simulink model "constant_volt"  (R2023b)
settings: Solver=VariableStepAuto  StartTime=0.0  StopTime=stepp.sim_time  RelTol=1e-3
values from neighbouring files (symbols this model uses):
  Bat =     [Samsung_30Q_18650_pack.mat]
undefined symbols (not defined in the file or in its folder): boost, ccm_m_op, ccm_reg_param, Ci, dcm_op, dcm_reg_param, Gp_ccm, Gp_dcm, Kr, m0_ccm, pv_data, pv_eq, Ramp, Ru, sim_op, stepp, Ti
libraries: spsSeriesRLCBranchLib x7, spsCurrentMeasurementLib x4, spsVoltageMeasurementLib x3, slpidlib x3, spsDiodeLib x1, spsControlledCurrentSourceLib x1, spsIdealSwitchLib x1, spsControlledVoltageSourceLib x1, simulink_extras x1, spsBistableLib x1, sps_lib x1
settings Model: Creator=teo  LastModifiedBy=teo
settings DataIOCC: ReturnWorkspaceOutputsName=CV_response

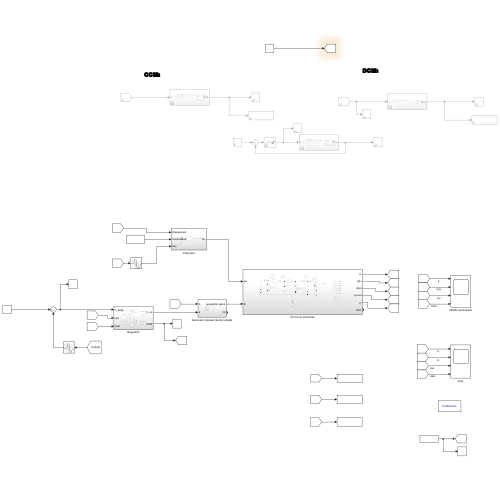
[thumbnail: Simulink's stored preview of the top-level diagram]
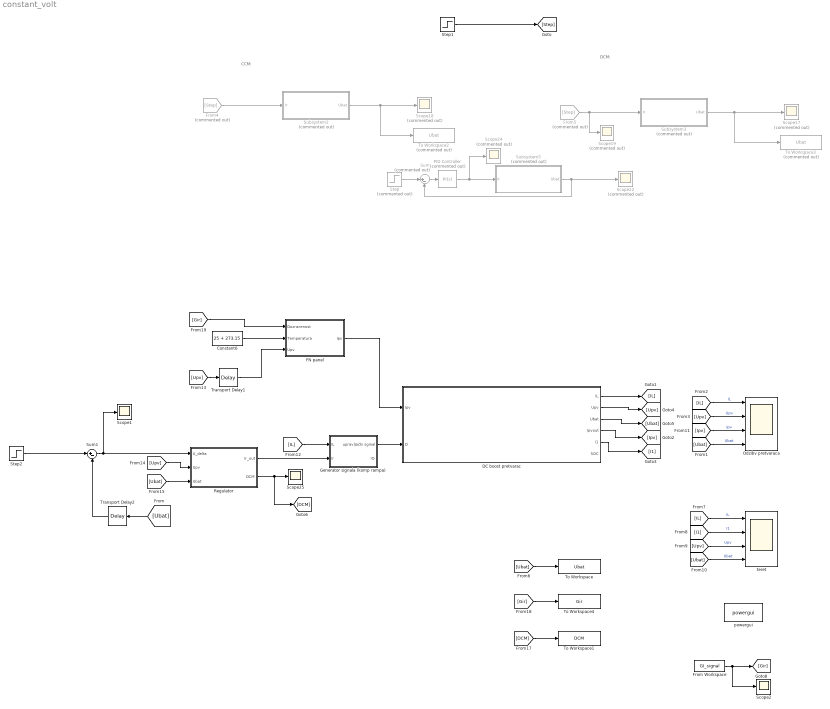
== system constant_volt ==
  note: CCM:
  note: DCM:
  Constant6 : Constant  Value=25 + 273.15
  DC boost pretvarac : Subsystem
  FN panel : Subsystem
  From Workspace : FromWorkspace  VariableName=GI_signal
  From4 : From  Commented=on  GotoTag=Step
  From5 : From  Commented=on  GotoTag=Step
  Generator signala (komp rampa) : Subsystem
  Odzibv pretvaraca : Scope  NumInputPorts=4
  PID Controller : slpidlib/PID Controller  Commented=on  Controller=PI  Form=Parallel  TimeDomain=Continuous-time  UseExternalTs=off  SampleTime=-1  IntegratorMethod=Forward Euler  FilterMethod=Forward Euler  ControllerParametersSource=internal  P=Kr  I=Kr/Ti  UseKiTs=off  D=0  N=100  UseFilter=on  TunerSelectOption=Transfer Function Based (PID Tuner App)  InitialConditionSource=internal  InitialConditionForIntegrator=0  InitialConditionForFilter=0  DifferentiatorICPrevScaledInput=0  ExternalReset=none  TrackingMode=off  Kt=1  LimitOutput=on  SatLimitsSource=internal  UpperSaturationLimit=2  LowerSaturationLimit=-2  LinearizeAsGain=off  AntiWindupMode=clamping  Kb=1  LimitIntegrator=off  UpperIntegratorSaturationLimit=inf  LowerIntegratorSaturationLimit=-inf  POutMin=[]  POutMax=[]  IOutMin=[]  IOutMax=[]  DOutMin=[]  DOutMax=[]  NOutMin=[]  NOutMax=[]  SumOutMin=[]  SumOutMax=[]  SaturationOutMin=[]  SaturationOutMax=[]  PParamMin=[]  PParamMax=[]  IParamMin=[]  IParamMax=[]  DParamMin=[]  DParamMax=[]  NParamMin=[]  NParamMax=[]  KbParamMin=[]  KbParamMax=[]  KtParamMin=[]  KtParamMax=[]  KbOutMin=[]  KbOutMax=[]  KtOutMin=[]  KtOutMax=[]  IntegratorOutMin=[]  IntegratorOutMax=[]  FilterOutMin=[]  FilterOutMax=[]  SumI1OutMin=[]  SumI1OutMax=[]  SumI2OutMin=[]  SumI2OutMax=[]  SumI3OutMin=[]  SumI3OutMax=[]  SumI4OutMin=[]  SumI4OutMax=[]  SumDOutMin=[]  SumDOutMax=[]  DifferentiatorOutMin=[]  DifferentiatorOutMax=[]  FilterDiffOutCoefMin=[]  FilterDiffOutCoefMax=[]  ReciprocalOutMin=[]  ReciprocalOutMax=[]  SumDenOutMin=[]  SumDenOutMax=[]  SumNumOutMin=[]  SumNumOutMax=[]  DivideOutMin=[]  DivideOutMax=[]  UdiffTsProdOutMin=[]  UdiffTsProdOutMax=[]  NTsProdOutMin=[]  NTsProdOutMax=[]  UintegralTsProdOutMin=[]  UintegralTsProdOutMax=[]  UngainTsProdOutMin=[]  UngainTsProdOutMax=[]  ClampingZeroOutDataTypeStr=Inherit: Inherit via back propagation  ClampingZeroOutMin=[]  ClampingZeroOutMax=[]  FilterDenConstantOutDataTypeStr=Inherit: Inherit via back propagation  FilterDenConstantOutMin=[]  FilterDenConstantOutMax=[]  PCopyOutDataTypeStr=Inherit: Inherit via back propagation  PCopyOutMin=[]  PCopyOutMax=[]  NCopyOutDataTypeStr=Inherit: Inherit via back propagation  NCopyOutMin=[]  NCopyOutMax=[]  IntegratorContinuousStateAttributes=''  IntegratorStateMustResolveToSignalObject=off  IntegratorRTWStateStorageClass=Auto  FilterContinuousStateAttributes=''  FilterStateMustResolveToSignalObject=off  FilterRTWStateStorageClass=Auto  ParallelPVariant=InternalParameters  IdealPVariant=Disabled  IVariant=InternalParameters  DVariant=Disabled  IntegratorVariant=Continuous  SatVariant=Enabled  AWVariant=ContClampingParallel  PCopyVariant=Disabled  TRVariant=Disabled  FdbkBlocksVariant=Forward  IdealPFdbkVariant=Disabled  SatFdbkVariant=Disabled  DerivativeFilterVariant=Disabled  NVariant=Disabled  NCopyVariant=Disabled_SignalSpec  FilterICVariant=Disabled  IntegratorICVariant=InternalICs  ExternalResetVariant=Disabled  TRSumVariant=Passthrough  SumFdbkVariant=Disabled  SumVariant=Sum_PI  TsampFilterVariant=InternalTs  TsampNgainVariant=Passthrough  TsampIntegralVariant=Disabled_SignalSpec  ExternalSaturationOutDataTypeStr=Inherit: Same as second input
  Regulator : Subsystem
  Scope1 : Scope
  Scope{17..19,22,24} (5 alike) : Scope  Commented=on
  Scope2 : Scope
  Scope25 : Scope
  Step : Step  Commented=on  Time=stepp.step_time  After=Bat.Ubat_charged - 2.6  SampleTime=0
  Step1 : Step  Time=stepp.step_time  Before=stepp.ir01  After=stepp.ir02  SampleTime=0
  Step2 : Step  Time=stepp.sim_time/2  Before=12.55  After=12.6  SampleTime=0
  Subsystem2 : Subsystem  Commented=on
  Subsystem3 : Subsystem  Commented=on
  Subsystem5 : Subsystem  Commented=on
  Sum : Sum  Commented=on  Inputs=|+-
  Sum1 : Sum  Inputs=|+-
  To Workspace : ToWorkspace  VariableName=Ubat  SaveFormat=Timeseries  SampleTime=-1
  To Workspace1 : ToWorkspace  VariableName=DCM  SaveFormat=Timeseries  SampleTime=-1
  To Workspace2 : ToWorkspace  Commented=on  VariableName=Ubat  SaveFormat=Timeseries  SampleTime=1e-6
  To Workspace3 : ToWorkspace  Commented=on  VariableName=Ubat  SaveFormat=Timeseries  SampleTime=1e-6
  To Workspace4 : ToWorkspace  VariableName=Gir  SaveFormat=Timeseries  SampleTime=-1
  Transport Delay1 : TransportDelay  DelayTime=0.0001  BufferSize=4024
  Transport Delay2 : TransportDelay  DelayTime=boost.Tmfc  InitialOutput=sim_op.Ubat0  BufferSize=4024
  powergui : sps_lib/powergui  Priority=1  SimulationMode=Continuous  SampleTime=50e-6  frequency=60  Iterations=50  frequencyindice=0  Pbase=100e6  ErrMax=1e-4  UnitsV=kV  UnitsW=MW  buscounter=0  FunctionMessages=off  echomessages=off  EnableUseOfTLC=off  CurrentSourceSwitches=off  DisableSnubberDevices=off  DisableRonSwitches=off  DisableVfSwitches=off  DisplayEquations=off  AutomaticDiscreteSolvers=off  SolverType=Tustin/Backward Euler (TBE)  Interpol=off  ExternalGateDelay=off  methode=off  Ts=100  x0status=blocks  SPID=on  SwTol=0  HookPort=off  NonlinearTolerance=1e-4  nMaxIteration=100  ContinueOnMaxIteration=off  RestoreLinks=warning  ResistiveCurrentMeasurement=off  Frange=[0:2:500]  Ylog=off  Xlog=on  ShowGrid=off  save=off  variable=ZData  structure=0  ZoomFFT=off  StartTime=0.0  cycles=1  DisplayStyle=1  fundamental=60  FreqAxis=off  MaxFrequency=1000  frequencyindicesteady=1  RmsSteady=1  display=off
  teret : Scope  NumInputPorts=4
  wires:
  From4/1 -> Subsystem2/1(Ir)
  Subsystem2/1(Ubat) -> Scope18/1, To Workspace2/1
  From5/1 -> Scope19/1, Subsystem3/1(Ir)
  Subsystem3/1(Ubat) -> To Workspace3/1, Scope17/1
  Step1/1 -> [Step]
  Sum/1 -> PID Controller/1
  Subsystem5/1(Ubat) -> Scope22/1, Sum/2
  Step/1 -> Sum/1
  PID Controller/1 -> Scope24/1, Subsystem5/1(Ir)
  Constant6/1 -> FN panel/2(Temperatura)
  Transport Delay1/1 -> FN panel/3(Upv)
  FN panel/1(Ipv) -> DC boost pretvarac/1(Ipv)
  Generator signala (komp rampa)/1(upravljački sginal) -> DC boost pretvarac/2(D)
  Sum1/1 -> Regulator/1(U_delta), Scope1/1
  [I1] -> teret/2  "I1"
  DC boost pretvarac/2(Upv) -> [Upv]
  [IL] -> teret/1  "IL"
  DC boost pretvarac/3(Ubat) -> [Ubat]
  DC boost pretvarac/4(Ipvout) -> [Ipv]
  DC boost pretvarac/1(IL) -> [IL]
  [Upv] -> Odzibv pretvaraca/2  "Upv"
  [Ubat] -> teret/4  "Ubat"
  DC boost pretvarac/5(I1) -> [I1]
  [IL] -> Odzibv pretvaraca/1  "IL"
  [Upv] -> teret/3  "Upv"
  [Ipv] -> Odzibv pretvaraca/3  "Ipv"
  [Ubat] -> Odzibv pretvaraca/4  "Ubat"
  [Ubat] -> Transport Delay2/1
  Transport Delay2/1 -> Sum1/2
  [IL] -> Generator signala (komp rampa)/1(IL)
  [Upv] -> Transport Delay1/1
  [Upv] -> Regulator/2(Upv)
  [Ubat] -> Regulator/3(Ubat)
  Regulator/2(DCM) -> [DCM], Scope25/1
  Regulator/1(Ir_out) -> Generator signala (komp rampa)/2(Ir)
  [Ubat] -> To Workspace/1
  [DCM] -> To Workspace1/1
  [Gir] -> To Workspace4/1
  From Workspace/1 -> Scope2/1, [Gir]
  [Gir] -> FN panel/1(Dozracenost)
  Step2/1 -> Sum1/1

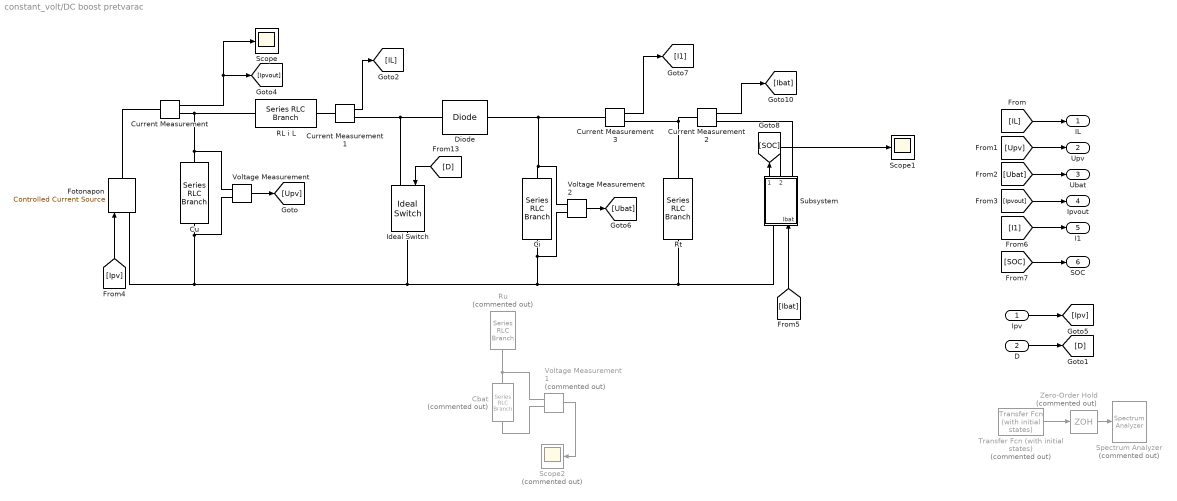
== system constant_volt/DC boost pretvarac ==
  Ipv : Inport
  D : Inport  Port=2
  Cbat : spsSeriesRLCBranchLib/Series RLC Branch  Commented=on  LConnTagsString=__new0  RConnTagsString=__new0  BranchType=C  Resistance=Ru  Inductance=1e-3  SetiL0=off  InitialCurrent=0  Capacitance=boost.Cbat  Setx0=on  InitialVoltage=sim_op.Ubat0  Measurements=None
  Ci : spsSeriesRLCBranchLib/Series RLC Branch  LConnTagsString=__new0  RConnTagsString=__new0  BranchType=C  Resistance=0.001  Inductance=1e-3  SetiL0=off  InitialCurrent=0  Capacitance=boost.Ci  Setx0=on  InitialVoltage=sim_op.Ubat0  Measurements=None
  Cu : spsSeriesRLCBranchLib/Series RLC Branch  LConnTagsString=__new0  RConnTagsString=__new0  BranchType=C  Resistance=0.001  Inductance=1e-3  SetiL0=off  InitialCurrent=0  Capacitance=boost.Cu  Setx0=on  InitialVoltage=sim_op.Upv0  Measurements=None
  Current Measurement{,1..3} (4 alike) : spsCurrentMeasurementLib/Current Measurement  PhasorSimulation=off  OutputType=Complex  PSBequivalent=0
  Diode : spsDiodeLib/Diode  Ron=0  Lon=0  Vf=0  IC=0  UseSnubber=0  Rs=0  Cs=0  Measurements=off
  Fotonapon : spsControlledCurrentSourceLib/Controlled Current Source  Initialize=on  Source_Type=DC  Amplitude=0  Phase=0  Frequency=0  Measurements=None
  Ideal Switch : spsIdealSwitchLib/Ideal Switch  Ron=0  Lon=0  IC=0  Rs=0  Cs=0  Measurements=off
  RL i L : spsSeriesRLCBranchLib/Series RLC Branch  LConnTagsString=__new0  RConnTagsString=__new0  BranchType=RL  Resistance=boost.RL  Inductance=boost.L  SetiL0=off  InitialCurrent=stepp.ir01  Capacitance=1e-6  Setx0=off  InitialVoltage=0  Measurements=None
  Rt : spsSeriesRLCBranchLib/Series RLC Branch  LConnTagsString=__new0  RConnTagsString=__new0  BranchType=R  Resistance=boost.Rt  Inductance=1e-3  SetiL0=off  InitialCurrent=0  Capacitance=Ci  Setx0=off  InitialVoltage=0  Measurements=None
  Ru : spsSeriesRLCBranchLib/Series RLC Branch  Commented=on  LConnTagsString=__new0  RConnTagsString=__new0  BranchType=R  Resistance=boost.Ru  Inductance=1e-3  SetiL0=off  InitialCurrent=0  Capacitance=Ci  Setx0=on  InitialVoltage=Ubat0_ccm  Measurements=None
  Scope : Scope
  Scope1 : Scope
  Scope2 : Scope  Commented=on
  Spectrum Analyzer : SpectrumAnalyzer  Commented=on  WindowPosition=[1.000000,1.000000,1920.000000,1080.000000,]  ScopeFrameLocation=window  Method=Welch  PlotAsTwoSidedSpectrum=off  Span=150000  CenterFrequency=75000  StartFrequency=0  StopFrequency=150000  AveragingMethod=Exponential  ForgettingFactor=1  YLimits=[-162.01370297,70.38685066]  ExpandToolstrip=on  SelectedToolstripTab=spectrumAnalyzerToolstrip.measurementsTab
  Subsystem : Subsystem
      settings: PortSchema="{\"entries\":[{\"content\":{\"sides\":[{\"content\":{\"connectorIds\":[\"LConn1\",\"In1\"]},\"type\":\"ConnectorPlacement.EquallySpacedRectSide\",\"uuid\":\"36a151cb-ade8-4d77-9227-5d94720a867f\"},{\"content\":{\"connectorIds\":[\"Out1\",\"Out2\",\"RConn1\"],\"side\":\"RIGHT\"},\"type\":\"ConnectorPlacement.EquallySpacedRectSide\",\"uuid\":\"e273b59b-5ac5-431a-9422-aa1eb85d6b42\"},{\"content\":{\"side\":\"TOP\"},\"type\":\"ConnectorPlacement.EquallySpacedRectSide\",\"uuid\":\"963da400-5a20-4c48-ad4c-e087b1b0be12\"}]},\"type\":\"ConnectorPlacement.EquallySpacedConnector\",\"uuid\":\"3f6c7281-abab-4595-a869-b172f12b4791\"}],\"packageUris\":[\"http://schema.mathworks.com/mf0/Connector/R2020b\"],\"version\":\"1.0\"}"
  Transfer Fcn (with initial states) : simulink_extras/Additional Linear/Transfer Fcn (with initial states)  Commented=on  N=[1]  D=[boost.Tmfc, 1]  X0=.5
  Voltage Measurement : spsVoltageMeasurementLib/Voltage Measurement  PhasorSimulation=off  OutputType=Complex  PSBequivalent=0
  Voltage Measurement1 : spsVoltageMeasurementLib/Voltage Measurement  Commented=on  PhasorSimulation=off  OutputType=Complex  PSBequivalent=0
  Voltage Measurement2 : spsVoltageMeasurementLib/Voltage Measurement  PhasorSimulation=off  OutputType=Complex  PSBequivalent=0
  Zero-Order Hold : ZeroOrderHold  Commented=on  SampleTime=1/(3*boost.f)
  IL : Outport
  Upv : Outport  Port=2
  Ubat : Outport  Port=3
  Ipvout : Outport  Port=4
  I1 : Outport  Port=5
  SOC : Outport  Port=6
  wires:
  Current Measurement1/1 -> [IL]
  Voltage Measurement/1 -> [Upv]
  [D] -> Ideal Switch/1
  [Ipv] -> Fotonapon/1
  D/1 -> [D]
  Ipv/1 -> [Ipv]
  [IL] -> IL/1
  [Upv] -> Upv/1
  [Ubat] -> Ubat/1
  Current Measurement/1 -> Scope/1, [Ipvout]
  [Ipvout] -> Ipvout/1
  [I1] -> I1/1
  Voltage Measurement1/1 -> Scope2/1
  Zero-Order Hold/1 -> Spectrum Analyzer/1
  Transfer Fcn (with initial states)/1 -> Zero-Order Hold/1
  Voltage Measurement2/1 -> [Ubat]
  Current Measurement2/1 -> [Ibat]
  [Ibat] -> Subsystem/1(Ibat)
  Subsystem/2(SOC) -> Scope1/1
  Current Measurement3/1 -> [I1]
  Subsystem/1(Uoc) -> [SOC]
  [SOC] -> SOC/1
  connections:
  Current Measurement/RConn1 -- Voltage Measurement/LConn1 -- Cu/LConn1 -- RL i L/LConn1
  RL i L/RConn1 -- Current Measurement1/LConn1
  Diode/LConn1 -- Ideal Switch/LConn1 -- Current Measurement1/RConn1
  Ci/RConn1 -- Voltage Measurement2/LConn2 -- Subsystem/LConn1 -- Rt/RConn1 -- Voltage Measurement/LConn2 -- Cu/RConn1 -- Fotonapon/LConn1 -- Ideal Switch/RConn1
  Fotonapon/RConn1 -- Current Measurement/LConn1
  Voltage Measurement2/LConn1 -- Current Measurement3/LConn1 -- Diode/RConn1 -- Ci/LConn1
  Ru/RConn1 -- Voltage Measurement1/LConn1 -- Cbat/LConn1
  Cbat/RConn1 -- Voltage Measurement1/LConn2
  Subsystem/RConn1 -- Current Measurement2/RConn1
  Rt/LConn1 -- Current Measurement3/RConn1 -- Current Measurement2/LConn1

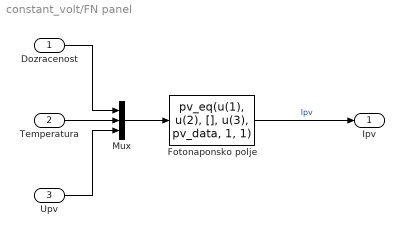
== system constant_volt/FN panel ==
  Dozracenost : Inport
  Temperatura : Inport  Port=2
  Upv : Inport  Port=3
  Fotonaponsko polje : MATLABFcn  MATLABFcn=pv_eq(u(1), u(2), [], u(3), pv_data, 1, 1)  OutputDimensions=1
  Mux : Mux  Inputs=3
  Ipv : Outport
  wires:
  Fotonaponsko polje/1 -> Ipv/1  "Ipv"
  Mux/1 -> Fotonaponsko polje/1
  Dozracenost/1 -> Mux/1
  Temperatura/1 -> Mux/2
  Upv/1 -> Mux/3

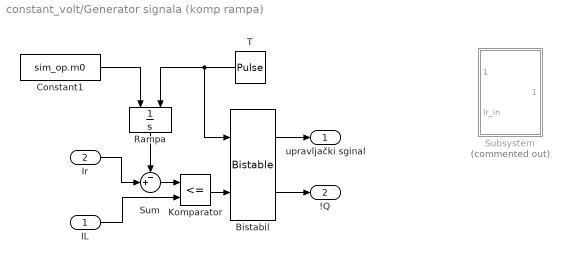
== system constant_volt/Generator signala (komp rampa) ==
  IL : Inport
  Ir : Inport  Port=2
  Bistabil : spsBistableLib/Bistable  Qpriority=Set  ic=0  Ts=0
      settings: LibrarySourceBlock=sps_lib/Control/Bistable
  Constant1 : Constant  Value=sim_op.m0
  Komparator : RelationalOperator  Operator=<=  OutDataTypeStr=boolean  RndMeth=Simplest  InputSameDT=off
  Rampa : Integrator  ExternalReset=rising
  Subsystem : Subsystem  Commented=on
  Sum : Sum  Inputs=-+|
  T : DiscretePulseGenerator  PulseType=Time based  Period=boost.T
  upravljački sginal : Outport
  !Q : Outport  Port=2
  wires:
  Komparator/1 -> Bistabil/2
  Bistabil/2 -> !Q/1
  Bistabil/1 -> upravljački sginal/1
  IL/1 -> Komparator/2
  Sum/1 -> Komparator/1
  Ir/1 -> Sum/2
  Rampa/1 -> Sum/1
  T/1 -> Bistabil/1, Rampa/2
  Constant1/1 -> Rampa/1

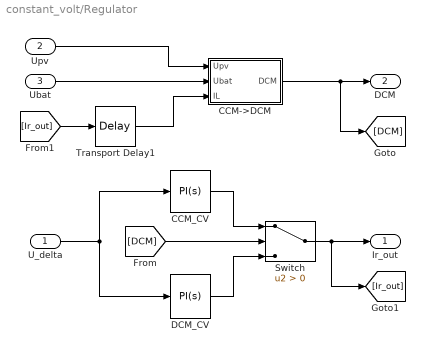
== system constant_volt/Regulator ==
  U_delta : Inport
  Upv : Inport  Port=2
  Ubat : Inport  Port=3
  CCM->DCM : Subsystem
  CCM_CV : slpidlib/PID Controller  Controller=PI  Form=Parallel  TimeDomain=Continuous-time  UseExternalTs=off  SampleTime=-1  IntegratorMethod=Forward Euler  FilterMethod=Forward Euler  ControllerParametersSource=internal  P=ccm_reg_param.KR  I=ccm_reg_param.KR/ccm_reg_param.Ti  UseKiTs=off  D=0  N=100  UseFilter=on  TunerSelectOption=Transfer Function Based (PID Tuner App)  InitialConditionSource=internal  InitialConditionForIntegrator=0  InitialConditionForFilter=0  DifferentiatorICPrevScaledInput=0  ExternalReset=none  TrackingMode=off  Kt=1  LimitOutput=on  SatLimitsSource=internal  UpperSaturationLimit=1.9  LowerSaturationLimit=-1.9  LinearizeAsGain=off  AntiWindupMode=clamping  Kb=1  LimitIntegrator=off  UpperIntegratorSaturationLimit=inf  LowerIntegratorSaturationLimit=-inf  POutMin=[]  POutMax=[]  IOutMin=[]  IOutMax=[]  DOutMin=[]  DOutMax=[]  NOutMin=[]  NOutMax=[]  SumOutMin=[]  SumOutMax=[]  SaturationOutMin=[]  SaturationOutMax=[]  PParamMin=[]  PParamMax=[]  IParamMin=[]  IParamMax=[]  DParamMin=[]  DParamMax=[]  NParamMin=[]  NParamMax=[]  KbParamMin=[]  KbParamMax=[]  KtParamMin=[]  KtParamMax=[]  KbOutMin=[]  KbOutMax=[]  KtOutMin=[]  KtOutMax=[]  IntegratorOutMin=[]  IntegratorOutMax=[]  FilterOutMin=[]  FilterOutMax=[]  SumI1OutMin=[]  SumI1OutMax=[]  SumI2OutMin=[]  SumI2OutMax=[]  SumI3OutMin=[]  SumI3OutMax=[]  SumI4OutMin=[]  SumI4OutMax=[]  SumDOutMin=[]  SumDOutMax=[]  DifferentiatorOutMin=[]  DifferentiatorOutMax=[]  FilterDiffOutCoefMin=[]  FilterDiffOutCoefMax=[]  ReciprocalOutMin=[]  ReciprocalOutMax=[]  SumDenOutMin=[]  SumDenOutMax=[]  SumNumOutMin=[]  SumNumOutMax=[]  DivideOutMin=[]  DivideOutMax=[]  UdiffTsProdOutMin=[]  UdiffTsProdOutMax=[]  NTsProdOutMin=[]  NTsProdOutMax=[]  UintegralTsProdOutMin=[]  UintegralTsProdOutMax=[]  UngainTsProdOutMin=[]  UngainTsProdOutMax=[]  ClampingZeroOutDataTypeStr=Inherit: Inherit via back propagation  ClampingZeroOutMin=[]  ClampingZeroOutMax=[]  FilterDenConstantOutDataTypeStr=Inherit: Inherit via back propagation  FilterDenConstantOutMin=[]  FilterDenConstantOutMax=[]  PCopyOutDataTypeStr=Inherit: Inherit via back propagation  PCopyOutMin=[]  PCopyOutMax=[]  NCopyOutDataTypeStr=Inherit: Inherit via back propagation  NCopyOutMin=[]  NCopyOutMax=[]  IntegratorContinuousStateAttributes=''  IntegratorStateMustResolveToSignalObject=off  IntegratorRTWStateStorageClass=Auto  FilterContinuousStateAttributes=''  FilterStateMustResolveToSignalObject=off  FilterRTWStateStorageClass=Auto  ParallelPVariant=InternalParameters  IdealPVariant=Disabled  IVariant=InternalParameters  DVariant=Disabled  IntegratorVariant=Continuous  SatVariant=Enabled  AWVariant=ContClampingParallel  PCopyVariant=Disabled  TRVariant=Disabled  FdbkBlocksVariant=Forward  IdealPFdbkVariant=Disabled  SatFdbkVariant=Disabled  DerivativeFilterVariant=Disabled  NVariant=Disabled  NCopyVariant=Disabled_SignalSpec  FilterICVariant=Disabled  IntegratorICVariant=InternalICs  ExternalResetVariant=Disabled  TRSumVariant=Passthrough  SumFdbkVariant=Disabled  SumVariant=Sum_PI  TsampFilterVariant=InternalTs  TsampNgainVariant=Passthrough  TsampIntegralVariant=Disabled_SignalSpec  ExternalSaturationOutDataTypeStr=Inherit: Same as second input
  DCM_CV : slpidlib/PID Controller  Controller=PI  Form=Parallel  TimeDomain=Continuous-time  UseExternalTs=off  SampleTime=-1  IntegratorMethod=Forward Euler  FilterMethod=Forward Euler  ControllerParametersSource=internal  P=dcm_reg_param.KR  I=dcm_reg_param.KR/dcm_reg_param.Ti  UseKiTs=off  D=0  N=100  UseFilter=on  TunerSelectOption=Transfer Function Based (PID Tuner App)  InitialConditionSource=internal  InitialConditionForIntegrator=0  InitialConditionForFilter=0  DifferentiatorICPrevScaledInput=0  ExternalReset=none  TrackingMode=off  Kt=1  LimitOutput=on  SatLimitsSource=internal  UpperSaturationLimit=1.9  LowerSaturationLimit=-1.9  LinearizeAsGain=off  AntiWindupMode=clamping  Kb=1  LimitIntegrator=off  UpperIntegratorSaturationLimit=inf  LowerIntegratorSaturationLimit=-inf  POutMin=[]  POutMax=[]  IOutMin=[]  IOutMax=[]  DOutMin=[]  DOutMax=[]  NOutMin=[]  NOutMax=[]  SumOutMin=[]  SumOutMax=[]  SaturationOutMin=[]  SaturationOutMax=[]  PParamMin=[]  PParamMax=[]  IParamMin=[]  IParamMax=[]  DParamMin=[]  DParamMax=[]  NParamMin=[]  NParamMax=[]  KbParamMin=[]  KbParamMax=[]  KtParamMin=[]  KtParamMax=[]  KbOutMin=[]  KbOutMax=[]  KtOutMin=[]  KtOutMax=[]  IntegratorOutMin=[]  IntegratorOutMax=[]  FilterOutMin=[]  FilterOutMax=[]  SumI1OutMin=[]  SumI1OutMax=[]  SumI2OutMin=[]  SumI2OutMax=[]  SumI3OutMin=[]  SumI3OutMax=[]  SumI4OutMin=[]  SumI4OutMax=[]  SumDOutMin=[]  SumDOutMax=[]  DifferentiatorOutMin=[]  DifferentiatorOutMax=[]  FilterDiffOutCoefMin=[]  FilterDiffOutCoefMax=[]  ReciprocalOutMin=[]  ReciprocalOutMax=[]  SumDenOutMin=[]  SumDenOutMax=[]  SumNumOutMin=[]  SumNumOutMax=[]  DivideOutMin=[]  DivideOutMax=[]  UdiffTsProdOutMin=[]  UdiffTsProdOutMax=[]  NTsProdOutMin=[]  NTsProdOutMax=[]  UintegralTsProdOutMin=[]  UintegralTsProdOutMax=[]  UngainTsProdOutMin=[]  UngainTsProdOutMax=[]  ClampingZeroOutDataTypeStr=Inherit: Inherit via back propagation  ClampingZeroOutMin=[]  ClampingZeroOutMax=[]  FilterDenConstantOutDataTypeStr=Inherit: Inherit via back propagation  FilterDenConstantOutMin=[]  FilterDenConstantOutMax=[]  PCopyOutDataTypeStr=Inherit: Inherit via back propagation  PCopyOutMin=[]  PCopyOutMax=[]  NCopyOutDataTypeStr=Inherit: Inherit via back propagation  NCopyOutMin=[]  NCopyOutMax=[]  IntegratorContinuousStateAttributes=''  IntegratorStateMustResolveToSignalObject=off  IntegratorRTWStateStorageClass=Auto  FilterContinuousStateAttributes=''  FilterStateMustResolveToSignalObject=off  FilterRTWStateStorageClass=Auto  ParallelPVariant=InternalParameters  IdealPVariant=Disabled  IVariant=InternalParameters  DVariant=Disabled  IntegratorVariant=Continuous  SatVariant=Enabled  AWVariant=ContClampingParallel  PCopyVariant=Disabled  TRVariant=Disabled  FdbkBlocksVariant=Forward  IdealPFdbkVariant=Disabled  SatFdbkVariant=Disabled  DerivativeFilterVariant=Disabled  NVariant=Disabled  NCopyVariant=Disabled_SignalSpec  FilterICVariant=Disabled  IntegratorICVariant=InternalICs  ExternalResetVariant=Disabled  TRSumVariant=Passthrough  SumFdbkVariant=Disabled  SumVariant=Sum_PI  TsampFilterVariant=InternalTs  TsampNgainVariant=Passthrough  TsampIntegralVariant=Disabled_SignalSpec  ExternalSaturationOutDataTypeStr=Inherit: Same as second input
  Switch : Switch  Criteria=u2 > Threshold  SaturateOnIntegerOverflow=off  InputSameDT=off
  Transport Delay1 : TransportDelay  DelayTime=0.0001  InitialOutput=sim_op.Ubat0  BufferSize=4024
  Ir_out : Outport
  DCM : Outport  Port=2
  wires:
  CCM_CV/1 -> Switch/1
  Upv/1 -> CCM->DCM/1(Upv)
  Ubat/1 -> CCM->DCM/2(Ubat)
  CCM->DCM/1(DCM) -> DCM/1, [DCM]
  [Ir_out] -> Transport Delay1/1
  Transport Delay1/1 -> CCM->DCM/3(IL)
  DCM_CV/1 -> Switch/3
  [DCM] -> Switch/2
  U_delta/1 -> DCM_CV/1, CCM_CV/1
  Switch/1 -> [Ir_out], Ir_out/1

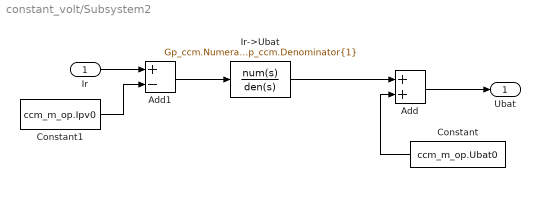
== system constant_volt/Subsystem2 ==
  Ir : Inport
  Add : Sum
  Add1 : Sum  Inputs=+-
  Constant : Constant  Value=ccm_m_op.Ubat0
  Constant1 : Constant  Value=ccm_m_op.Ipv0
  Ir->Ubat : TransferFcn  Numerator=Gp_ccm.Numerator{1}  Denominator=Gp_ccm.Denominator{1}
  Ubat : Outport
  wires:
  Ir/1 -> Add1/1
  Constant1/1 -> Add1/2
  Add1/1 -> Ir->Ubat/1
  Add/1 -> Ubat/1
  Constant/1 -> Add/2
  Ir->Ubat/1 -> Add/1

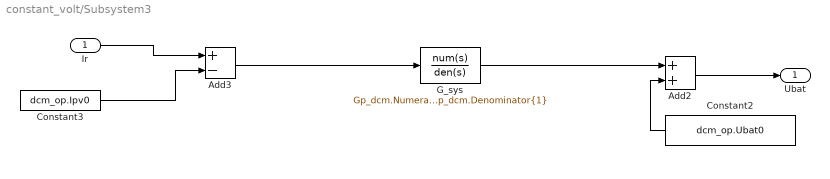
== system constant_volt/Subsystem3 ==
  Ir : Inport
  Add2 : Sum
  Add3 : Sum  Inputs=+-
  Constant2 : Constant  Value=dcm_op.Ubat0
  Constant3 : Constant  Value=dcm_op.Ipv0
  G_sys : TransferFcn  Numerator=Gp_dcm.Numerator{1}  Denominator=Gp_dcm.Denominator{1}
  Ubat : Outport
  wires:
  Constant3/1 -> Add3/2
  Add3/1 -> G_sys/1
  G_sys/1 -> Add2/1
  Constant2/1 -> Add2/2
  Ir/1 -> Add3/1
  Add2/1 -> Ubat/1

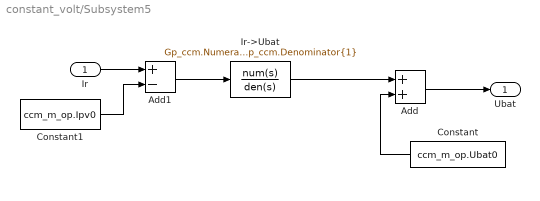
== system constant_volt/Subsystem5 ==
  Ir : Inport
  Add : Sum
  Add1 : Sum  Inputs=+-
  Constant : Constant  Value=ccm_m_op.Ubat0
  Constant1 : Constant  Value=ccm_m_op.Ipv0
  Ir->Ubat : TransferFcn  Numerator=Gp_ccm.Numerator{1}  Denominator=Gp_ccm.Denominator{1}
  Ubat : Outport
  wires:
  Ir/1 -> Add1/1
  Constant1/1 -> Add1/2
  Add1/1 -> Ir->Ubat/1
  Add/1 -> Ubat/1
  Constant/1 -> Add/2
  Ir->Ubat/1 -> Add/1

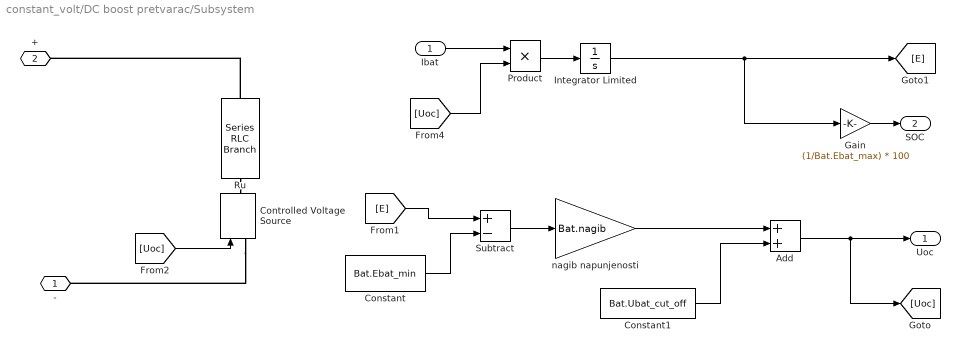
== system constant_volt/DC boost pretvarac/Subsystem ==
  Ibat : Inport
  Add : Sum
  Constant : Constant  Value=Bat.Ebat_min
  Constant1 : Constant  Value=Bat.Ubat_cut_off
  Controlled Voltage Source : spsControlledVoltageSourceLib/Controlled Voltage Source  Initialize=on  Source_Type=DC  Amplitude=sim_op.Ubat0  Phase=0  Frequency=0  Measurements=None
  Gain : Gain  Gain=(1/Bat.Ebat_max) * 100
  Integrator Limited : Integrator  InitialCondition=sim_op.E0  LimitOutput=on  UpperSaturationLimit=Bat.Ebat_max  LowerSaturationLimit=Bat.Ebat_min
  Product : Product
  Ru : spsSeriesRLCBranchLib/Series RLC Branch  LConnTagsString=__new0  RConnTagsString=__new0  BranchType=R  Resistance=boost.Ru  Inductance=1e-3  SetiL0=off  InitialCurrent=0  Capacitance=Ci  Setx0=off  InitialVoltage=0  Measurements=None
  Subtract : Sum  Inputs=+-
  nagib napunjenosti : Gain  Gain=Bat.nagib
  - : PMIOPort  Side=Left
  + : PMIOPort  Port=2  Side=Right
  Uoc : Outport
  SOC : Outport  Port=2
  wires:
  Subtract/1 -> nagib napunjenosti/1
  Constant/1 -> Subtract/2
  nagib napunjenosti/1 -> Add/1
  Constant1/1 -> Add/2
  Integrator Limited/1 -> Gain/1, [E]
  [Uoc] -> Product/2
  Product/1 -> Integrator Limited/1
  Ibat/1 -> Product/1
  [E] -> Subtract/1
  [Uoc] -> Controlled Voltage Source/1
  Gain/1 -> SOC/1
  Add/1 -> Uoc/1, [Uoc]
  connections:
  Controlled Voltage Source/LConn1 -- -/RConn1
  Ru/RConn1 -- Controlled Voltage Source/RConn1
  Ru/LConn1 -- +/RConn1

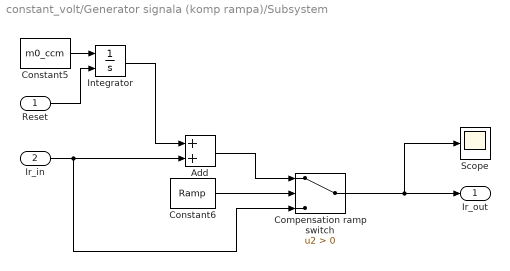
== system constant_volt/Generator signala (komp rampa)/Subsystem ==
  Reset : Inport
  Ir_in : Inport  Port=2
  Add : Sum
  Compensation ramp switch : Switch  Criteria=u2 > Threshold  SaturateOnIntegerOverflow=off  InputSameDT=off
  Constant5 : Constant  Value=m0_ccm
  Constant6 : Constant  Value=Ramp
  Integrator : Integrator  ExternalReset=rising
  Scope : Scope
  Ir_out : Outport
  wires:
  Constant5/1 -> Integrator/1
  Integrator/1 -> Add/1
  Add/1 -> Compensation ramp switch/1
  Reset/1 -> Integrator/2
  Compensation ramp switch/1 -> Scope/1, Ir_out/1
  Constant6/1 -> Compensation ramp switch/2
  Ir_in/1 -> Compensation ramp switch/3, Add/2

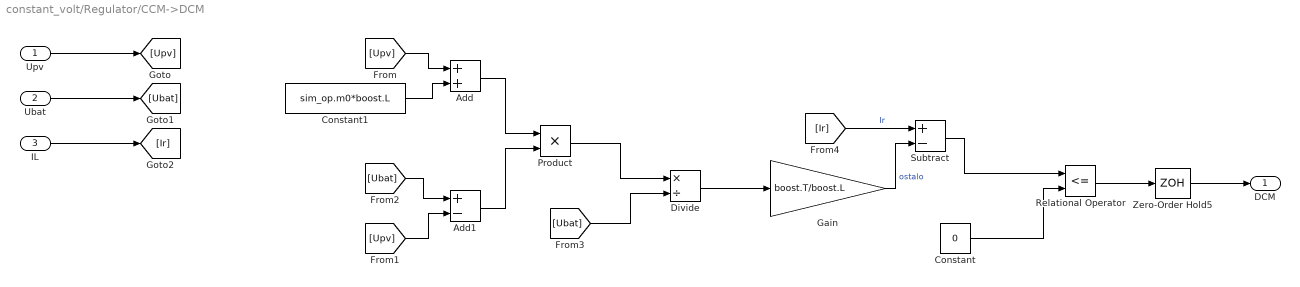
== system constant_volt/Regulator/CCM->DCM ==
  Upv : Inport
  Ubat : Inport  Port=2
  IL : Inport  Port=3
  Add : Sum
  Add1 : Sum  Inputs=+-
  Constant : Constant  Value=0
  Constant1 : Constant  Value=sim_op.m0*boost.L
  Divide : Product  Inputs=*/
  Gain : Gain  Gain=boost.T/boost.L
  Product : Product
  Relational Operator : RelationalOperator  Operator=<=  OutDataTypeStr=boolean  RndMeth=Simplest  InputSameDT=off
  Subtract : Sum  Inputs=+-
  Zero-Order Hold5 : ZeroOrderHold  SampleTime=0.002
  DCM : Outport
  wires:
  Product/1 -> Divide/1
  Constant1/1 -> Add/2
  Add/1 -> Product/1
  Add1/1 -> Product/2
  Divide/1 -> Gain/1
  [Upv] -> Add/1
  [Upv] -> Add1/2
  [Ubat] -> Add1/1
  [Ubat] -> Divide/2
  Gain/1 -> Subtract/2  "ostalo"
  [Ir] -> Subtract/1  "Ir"
  Constant/1 -> Relational Operator/2
  Upv/1 -> [Upv]
  Ubat/1 -> [Ubat]
  IL/1 -> [Ir]
  Relational Operator/1 -> Zero-Order Hold5/1
  Zero-Order Hold5/1 -> DCM/1
  Subtract/1 -> Relational Operator/1
